simulink model "Simulink_PID_Cascata"  (R2025b)
settings: Solver=VariableStepAuto  StartTime=0.0  StopTime=10.0  RelTol=1e-3
InitFcn:
  | run("init.m");
StopFcn:
  | run("video.m");
values from neighbouring files (symbols this model uses):
  q0_guess = [pi/3; -pi/6; pi/3]    [init.m]
undefined symbols (not defined in the file or in its folder): robot_params
settings Model: Creator=Acer  LastModifiedBy=Acer

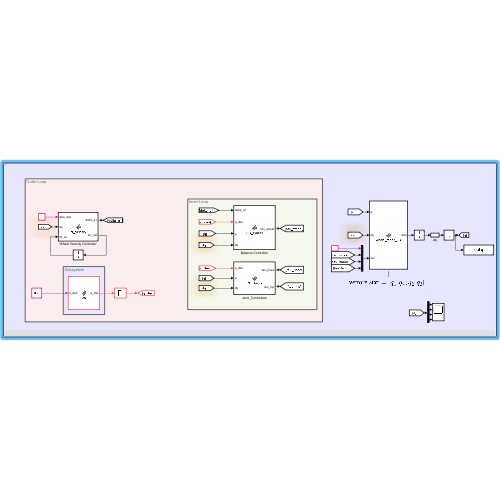
[thumbnail: Simulink's stored preview of the top-level diagram]
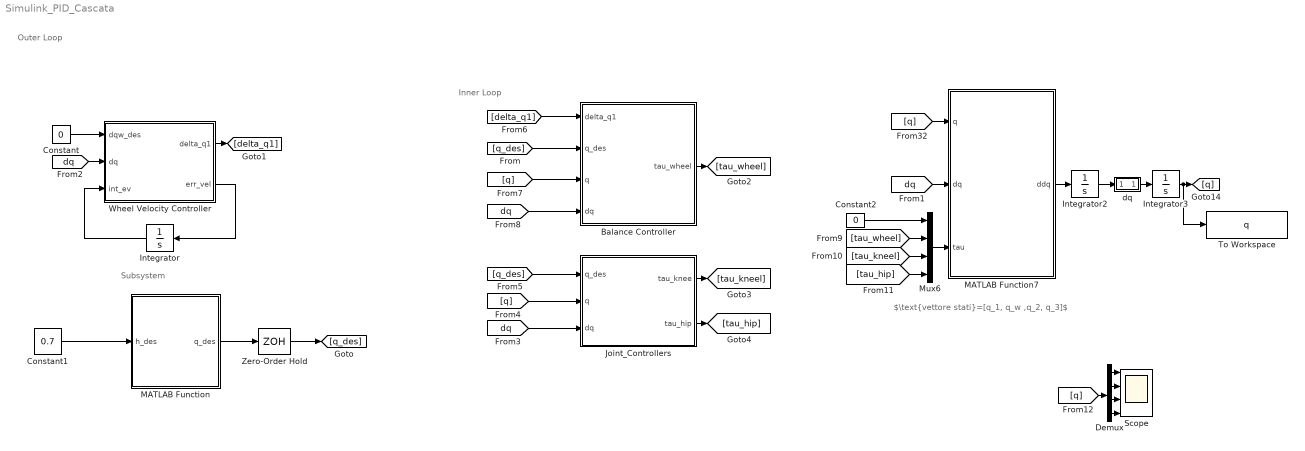
== system Simulink_PID_Cascata ==
  note: $\text{vettore stati}=[q_1, q_w ,q_2, q_3]$
  note: Subsystem
  note: Inner Loop
  note: Outer Loop
  Balance Controller : MATLAB Function  TreatAsAtomicUnit=on
  Constant : Constant  Value=0
  Constant1 : Constant  Value=0.7
  Constant2 : Constant  Value=0
  Demux : Demux
  Integrator : Integrator
  Integrator2 : Integrator  InitialCondition=zeros(4,1)
  Integrator3 : Integrator  InitialCondition=[q0_guess(1);0;q0_guess(2);q0_guess(3)]
  Joint_Controllers : MATLAB Function  TreatAsAtomicUnit=on
  MATLAB Function : MATLAB Function  TreatAsAtomicUnit=on
  MATLAB Function7 : MATLAB Function  TreatAsAtomicUnit=on
  Mux6 : Mux
  Scope : Scope  NumInputPorts=4
      settings: ActiveDisplayYMinimum=0.81487813935275555  ActiveDisplayYMaximum=3.1380722577911779
  To Workspace : ToWorkspace  VariableName=q  SaveFormat=Timeseries  SampleTime=-1
  Wheel Velocity Controller : MATLAB Function  TreatAsAtomicUnit=on
  Zero-Order Hold : ZeroOrderHold  SampleTime=-1
  dq : Subsystem
  wires:
  Mux6/1 -> MATLAB Function7/3(tau)
  [q] -> MATLAB Function7/1(q)
  Integrator3/1 -> To Workspace/1, [q]
  MATLAB Function7/1(ddq) -> Integrator2/1
  [dq] -> MATLAB Function7/2(dq)
  Constant/1 -> Wheel Velocity Controller/1(dqw_des)
  [dq] -> Wheel Velocity Controller/2(dq)
  Integrator2/1 -> dq/1(In1)
  dq/1(Out1) -> Integrator3/1
  [dq] -> Joint_Controllers/3(dq)
  [q] -> Joint_Controllers/2(q)
  [q_des] -> Balance Controller/2(q_des)
  [q_des] -> Joint_Controllers/1(q_des)
  Wheel Velocity Controller/1(delta_q1) -> [delta_q1]
  [delta_q1] -> Balance Controller/1(delta_q1)
  [q] -> Balance Controller/3(q)
  [dq] -> Balance Controller/4(dq)
  Wheel Velocity Controller/2(err_vel) -> Integrator/1
  Integrator/1 -> Wheel Velocity Controller/3(int_ev)
  MATLAB Function/1(q_des) -> Zero-Order Hold/1
  Constant1/1 -> MATLAB Function/1(h_des)
  Balance Controller/1(tau_wheel) -> [tau_wheel]
  Joint_Controllers/1(tau_knee) -> [tau_kneel]
  Joint_Controllers/2(tau_hip) -> [tau_hip]
  [tau_wheel] -> Mux6/2
  [tau_kneel] -> Mux6/3
  [tau_hip] -> Mux6/4
  Demux/2 -> Scope/2
  Demux/1 -> Scope/1
  Demux/3 -> Scope/3
  Demux/4 -> Scope/4
  [q] -> Demux/1
  Constant2/1 -> Mux6/1
  Zero-Order Hold/1 -> [q_des]

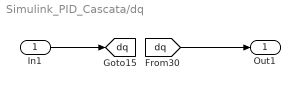
== system Simulink_PID_Cascata/dq ==
  In1 : Inport
  Out1 : Outport
  tag scope: dq=global
  wires:
  In1/1 -> [dq]
  [dq] -> Out1/1

== matlab function Simulink_PID_Cascata/Balance Controller ==
  data: delta_q1 input; tau_wheel output; q_des input; q input; dq input
function tau_wheel = PD_Wheel(delta_q1, q_des, q, dq)

% Il target reale dello stinco è ora modificato dal loop di velocità!
    q1_target_new = q_des(1) + delta_q1; 
    
    Kp_w = 400;  % Guadagno proporzionale ruota
    Kd_w = 80;   % Guadagno derivativo ruota
    
    e1 = q1_target_new - q(1);
    de1 = 0 - dq(1);
    
    % Generazione coppia di bilanciamento
    tau_wheel = Kp_w * e1 + Kd_w * de1;

== matlab function Simulink_PID_Cascata/Wheel Velocity Controller ==
  data: dqw_des input; delta_q1 output; dq input; int_ev input; err_vel output
function [delta_q1, err_vel] = PI_Velocity(dqw_des, dq, int_ev)

    % dqw_des velocita di riferimento della ruota
    
    err_vel = dqw_des - dq(2); % Errore di velocità della ruota
    
    % Guadagni PI (relativamente piccoli perché mappano velocità in radianti di inclinazione)
    Kp_v = 0.08; 
    Ki_v = 0.06;

    % L'output del loop di velocità è un "Angle Offset" (delta_q1)
    delta_q1 = -(Kp_v * err_vel + Ki_v * int_ev);

    % Saturazione di sicurezza per evitare che l'offset richieda inclinazioni estreme
    delta_q1 = max(min(delta_q1, 0.2), -0.2);

== matlab function Simulink_PID_Cascata/Joint_Controllers ==
  data: q_des input; tau_knee output; q input; tau_hip output; dq input
function [tau_knee, tau_hip] = PD_Joints(q_des, q, dq)

    Kp_j = 800; 
    Kd_j = 50;  
    
    e2 = q_des(2) - q(3);
    de2 = 0 - dq(3);
    tau_knee = Kp_j * e2 + Kd_j * de2;
    
    e3 = q_des(3) - q(4);
    de3 = 0 - dq(4);
    tau_hip = Kp_j * e3 + Kd_j * de3;

== matlab function Simulink_PID_Cascata/MATLAB Function ==
  settings: updateMethod=DISCRETE  sampleTime=0.1
  data: h_des input; q_des output; robot_params parameter; q0_guess parameter
function q_des = fcn(h_des, robot_params, q0_guess)
    % 1. Pre-allocazione per dire a Simulink che uscirà un vettore 3x1
    q_des = zeros(3,1);
    
    % 2. Dichiara la TUA funzione esterna come estrinseca (non fsolve)
    coder.extrinsic('calcola_target_cinematici');
    
    % 3. Inizializza la variabile temporanea per aiutare il Coder con i tipi
    q_des_calc = zeros(3,1);
    
    % 4. Richiama la funzione (il calcolo viene "appaltato" a MATLAB)
    q_des_calc = calcola_target_cinematici(h_des, robot_params, q0_guess);
    
    % 5. Assegnazione sicura all'uscita
    if ~isempty(q_des_calc)
        q_des = q_des_calc;
    end
end

== matlab function Simulink_PID_Cascata/MATLAB Function7 ==
  data: q input; ddq output size=4; dq input; tau input
function ddq =  whole_robot_2D(q, dq, tau)
    % tau è il vettore delle coppie/forze generalizzate in ingresso (4x1)
    
    [M, CdQ, G] = calc_dynamics(q, dq);

    %% equazione del moto: M*ddq + C*dq + G = tau
    % In MATLAB/Simulink si usa l'operatore mldivide (\) per invertire M in modo robusto
    ddq = M \ (tau - CdQ - G);
end
